simulink model "Lapsim3"  (R2020a)
settings: Solver=FixedStepAuto  StartTime=0.0  StopTime=t  FixedStep=0.01  RelTol=1e-3
values from neighbouring files (symbols this model uses):
  Ap = A + B*[k1 k2 k3]    [Lapunow.m]
  B = [0 ; 0 ; 50]    [Lapunow.m]
settings Model: Creator=SARIS  LastModifiedBy=grzyb

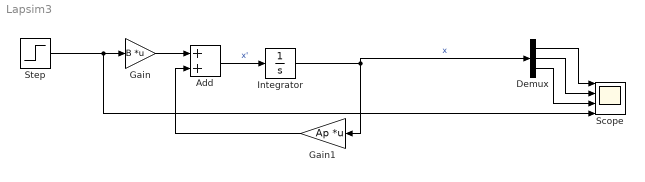
== system Lapsim3 ==
  Add : Sum
  Demux : Demux  Outputs=3
  Gain : Gain  Gain=B  Multiplication=Matrix(K*u)
  Gain1 : Gain  Gain=Ap  Multiplication=Matrix(K*u)
  Integrator : Integrator  InitialCondition=[0 0 0]
  Scope : Scope  NumInputPorts=4
  Step : Step  SampleTime=0
  wires:
  Gain/1 -> Add/1
  Add/1 -> Integrator/1  "x'"
  Gain1/1 -> Add/2
  Integrator/1 -> Demux/1, Gain1/1  "x"
  Demux/1 -> Scope/1
  Demux/2 -> Scope/2
  Demux/3 -> Scope/3
  Step/1 -> Scope/4, Gain/1
